simulink model "Gas_Turbine"  (R2023b)
settings: Solver=ode23t  StartTime=0.0  StopTime=30  RelTol=1e-3
settings Model: Creator=pmout  LastModifiedBy=pmout

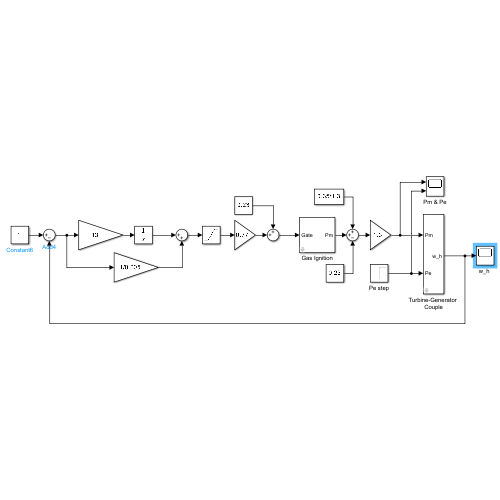
[thumbnail: Simulink's stored preview of the top-level diagram]
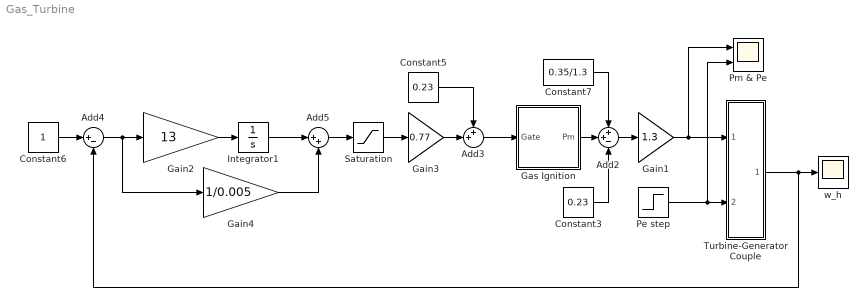
== system Gas_Turbine ==
  Add2 : Sum  Inputs=++-
  Add3 : Sum  Inputs=++|
  Add4 : Sum  Inputs=|+-
  Add5 : Sum  Inputs=|++
  Constant3 : Constant  Value=0.23
  Constant5 : Constant  Value=0.23
  Constant6 : Constant
  Constant7 : Constant  Value=0.35/1.3
  Gain1 : Gain  Gain=1.3
  Gain2 : Gain  Gain=13
  Gain3 : Gain  Gain=0.77
  Gain4 : Gain  Gain=1/0.005
  Gas Ignition : Subsystem  mask{Tw=0.4, ini=0.23+0.35/1.3}
      mask prompts: Tw "Gas ignition constant"; ini "Initial Pm"
  Integrator1 : Integrator
  Pe step : Step  Time=2  Before=0.35  After=0.55  SampleTime=0
  Pm & Pe : Scope  NumInputPorts=2
  Saturation : Saturate  UpperLimit=0.8  LowerLimit=-0.8
  Turbine-Generator Couple : Subsystem  mask{Hh=3.5, w_ini=1}
      mask prompts: Hh "H/E Inertia Constant"; w_ini "Initial omega"
  "w_h " : Scope
  wires:
  Constant5/1 -> Add3/1
  Gain4/1 -> Add5/2
  Add4/1 -> Gain4/1, Gain2/1
  Gain3/1 -> Add3/2
  Gain2/1 -> Integrator1/1
  Add2/1 -> Gain1/1
  Gain1/1 -> Pm & Pe/1, Turbine-Generator Couple/1(Pm)
  Constant6/1 -> Add4/1
  Gas Ignition/1(Pm) -> Add2/2
  Add5/1 -> Saturation/1
  Pe step/1 -> Pm & Pe/2, Turbine-Generator Couple/2(Pe)
  Integrator1/1 -> Add5/1
  Constant3/1 -> Add2/3
  Constant7/1 -> Add2/1
  Add3/1 -> Gas Ignition/1(Gate)
  Saturation/1 -> Gain3/1
  Turbine-Generator Couple/1(w_h) -> Add4/2, "w_h "/1

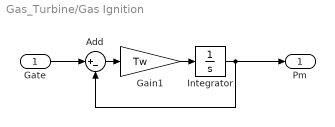
== system Gas_Turbine/Gas Ignition ==
  Gate : Inport
  Add : Sum  Inputs=|+-
  Gain1 : Gain  Gain=Tw
  Integrator : Integrator  InitialCondition=0.23
  Pm : Outport
  wires:
  Gain1/1 -> Integrator/1
  Add/1 -> Gain1/1
  Integrator/1 -> Pm/1, Add/2
  Gate/1 -> Add/1

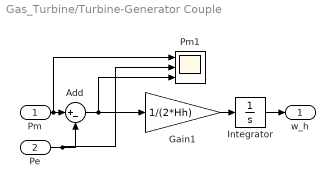
== system Gas_Turbine/Turbine-Generator Couple ==
  Pm : Inport
  Pe : Inport  Port=2
  Add : Sum  Inputs=|+-
  Gain1 : Gain  Gain=1/(2*Hh)
  Integrator : Integrator  InitialCondition=w_ini
  Pm1 : Scope  NumInputPorts=3
  w_h : Outport
  wires:
  Add/1 -> Gain1/1, Pm1/3
  Pe/1 -> Add/2, Pm1/2
  Integrator/1 -> w_h/1
  Gain1/1 -> Integrator/1
  Pm/1 -> Add/1, Pm1/1
